simulink model "rlLKAMdl"  (R2019a)
settings: Solver=VariableStepAuto  StartTime=0.0  StopTime=T  RelTol=1e-3
undefined symbols (not defined in the file): Cf, Cr, DiscIntNeverNeededParam, e1_initial, e2_initial, Iz, lf, lr, m, rho, Ts, u_max, u_min, Vx
libraries: rllib x1, simulink x1
settings Model: Creator=The MathWorks, Inc.  LastModifiedBy=The MathWorks, Inc.
settings DataIOCC: ReturnWorkspaceOutputs=off
settings DebuggingCC: ArithmeticOperatorsInVariantConditions=warning
settings SFSimCC: SimUseLocalCustomCode=off
settings RTWCC: RTWUseLocalCustomCode=off
settings CodeAppCC: StateflowObjectComments=on
settings SimscapeCC: SimscapeNormalizeSystem=off

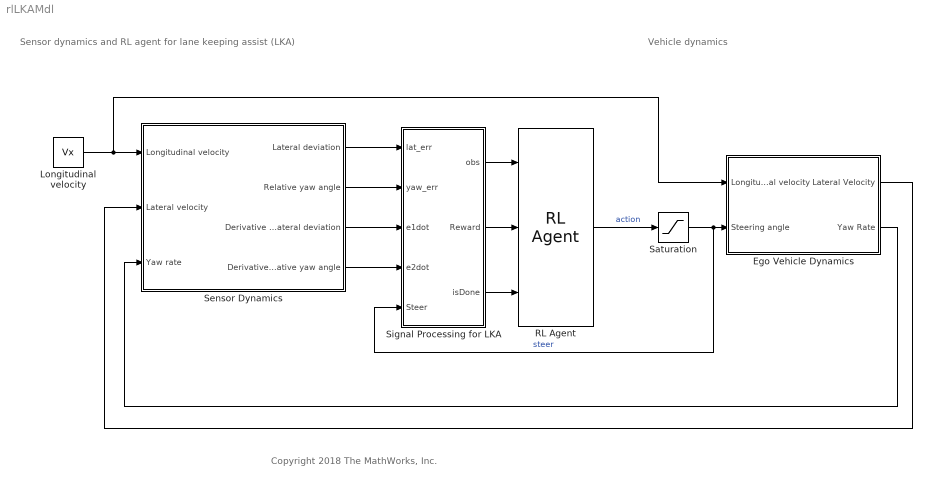
== system rlLKAMdl ==
  note: Vehicle dynamics
  note: Sensor dynamics and RL agent for lane keeping assist (LKA)
  note: Copyright 2018 The MathWorks, Inc.
  Ego Vehicle Dynamics : Subsystem
  Longitudinal velocity : Constant  Value=Vx  SampleTime=Ts
  RL Agent : rllib/RL Agent  Agent=agent  ProvideReward=on  ProvideIsDone=on  ProvideCumRwd=off  TreatAsDirectFeedthrough=on  CollectLoggedSignals=on  CollectModelStates=on
      settings: SourceProductName=Reinforcement Learning Toolbox
  Saturation : Saturate  UpperLimit=u_max  LowerLimit=u_min
  Sensor Dynamics : Subsystem
  "Signal Processing for LKA " : Subsystem
  wires:
  Ego Vehicle Dynamics/2(Yaw Rate) -> Sensor Dynamics/3(Yaw rate)
  Ego Vehicle Dynamics/1(Lateral Velocity) -> Sensor Dynamics/2(Lateral velocity)
  Longitudinal velocity/1 -> Sensor Dynamics/1(Longitudinal velocity), Ego Vehicle Dynamics/1(Longitudinal velocity)
  RL Agent/1 -> Saturation/1  "action"
  Saturation/1 -> "Signal Processing for LKA "/5(Steer), Ego Vehicle Dynamics/2(Steering angle)  "steer"
  Sensor Dynamics/1(Lateral deviation) -> "Signal Processing for LKA "/1(lat_err)
  Sensor Dynamics/2(Relative yaw angle) -> "Signal Processing for LKA "/2(yaw_err)
  "Signal Processing for LKA "/1(obs) -> RL Agent/1
  "Signal Processing for LKA "/2(Reward) -> RL Agent/2
  "Signal Processing for LKA "/3(isDone) -> RL Agent/3
  Sensor Dynamics/3(Derivative of lateral deviation) -> "Signal Processing for LKA "/3("e1dot ")
  Sensor Dynamics/4(Derivative of relative yaw angle) -> "Signal Processing for LKA "/4(e2dot)

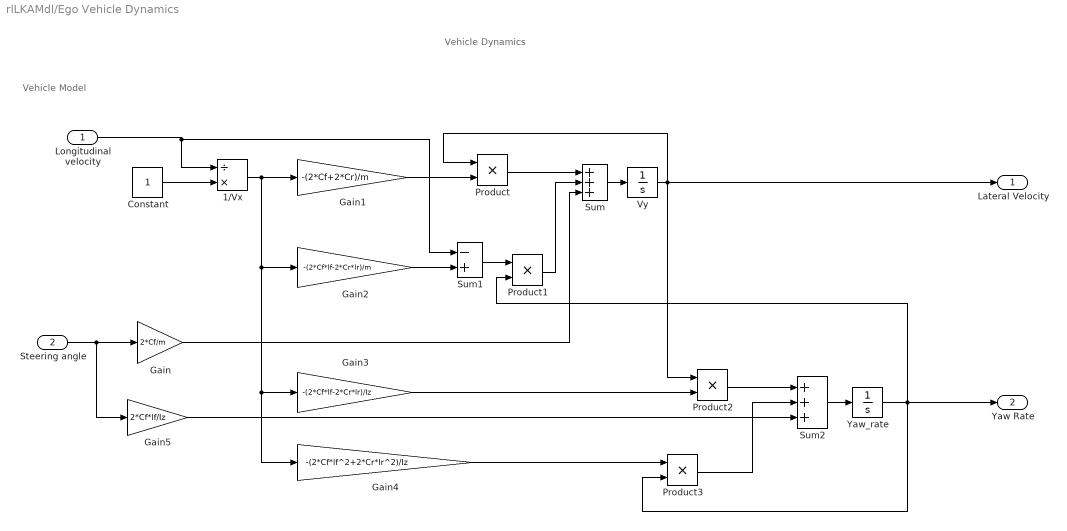
== system rlLKAMdl/Ego Vehicle Dynamics ==
  note: Vehicle Model
  note: Vehicle Dynamics
  Longitudinal velocity : Inport
  Steering angle : Inport  Port=2
  1/Vx : Product  Inputs=/*
  Constant : Constant
  Gain : Gain  Gain=2*Cf/m
  Gain1 : Gain  Gain=-(2*Cf+2*Cr)/m
  Gain2 : Gain  Gain=-(2*Cf*lf-2*Cr*lr)/m
  Gain3 : Gain  Gain=-(2*Cf*lf-2*Cr*lr)/Iz
  Gain4 : Gain  Gain=-(2*Cf*lf^2+2*Cr*lr^2)/Iz
  Gain5 : Gain  Gain=2*Cf*lf/Iz
  Product{,1..3} (4 alike) : Product
  Sum : Sum  Inputs=+++
  Sum1 : Sum  Inputs=-+
  Sum2 : Sum  Inputs=+++
  Vy : Integrator
  "Yaw_rate " : Integrator
  Lateral Velocity : Outport
  Yaw Rate : Outport  Port=2
  wires:
  Sum2/1 -> "Yaw_rate "/1
  Gain2/1 -> Sum1/2
  Gain4/1 -> Product3/1
  Constant/1 -> 1/Vx/2
  Gain3/1 -> Product2/2
  1/Vx/1 -> Gain4/1, Gain3/1, Gain2/1, Gain1/1
  Product2/1 -> Sum2/1
  Product3/1 -> Sum2/2
  Gain5/1 -> Sum2/3
  Sum1/1 -> Product1/1
  "Yaw_rate "/1 -> Product3/2, Yaw Rate/1, Product1/2
  Gain/1 -> Sum/3
  Steering angle/1 -> Gain/1, Gain5/1
  Gain1/1 -> Product/2
  Product/1 -> Sum/1
  Vy/1 -> Product/1, Lateral Velocity/1, Product2/1
  Sum/1 -> Vy/1
  Longitudinal velocity/1 -> Sum1/1, 1/Vx/1
  Product1/1 -> Sum/2

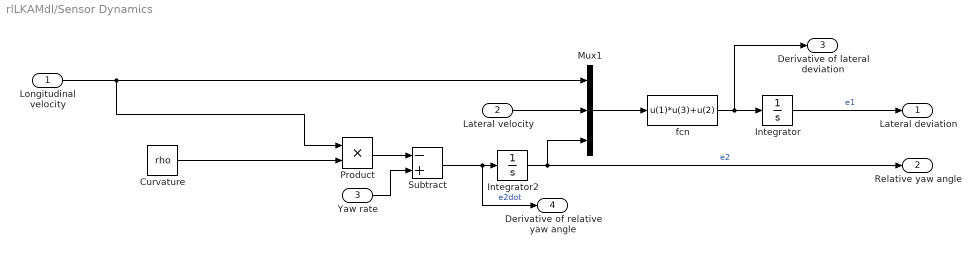
== system rlLKAMdl/Sensor Dynamics ==
  Longitudinal velocity : Inport
  Lateral velocity : Inport  Port=2
  Yaw rate : Inport  Port=3
  Curvature : Constant  Value=rho
  Integrator : Integrator  InitialCondition=e1_initial
  Integrator2 : Integrator  InitialCondition=e2_initial
  Mux1 : Mux  Inputs=[1 1 1]
  Product : Product
  Subtract : Sum  Inputs=-+
  fcn : Fcn  Expr=u(1)*u(3)+u(2)
  Lateral deviation : Outport
  Relative yaw angle : Outport  Port=2
  Derivative of lateral deviation : Outport  Port=3
  Derivative of relative yaw angle : Outport  Port=4
  wires:
  Integrator2/1 -> Relative yaw angle/1, Mux1/3  "e2"
  Mux1/1 -> fcn/1
  fcn/1 -> Derivative of lateral deviation/1, Integrator/1
  Lateral velocity/1 -> Mux1/2
  Integrator/1 -> Lateral deviation/1  "e1"
  Product/1 -> Subtract/1
  Yaw rate/1 -> Subtract/2
  Subtract/1 -> Derivative of relative yaw angle/1, Integrator2/1  "e2dot"
  Longitudinal velocity/1 -> Mux1/1, Product/1
  Curvature/1 -> Product/2

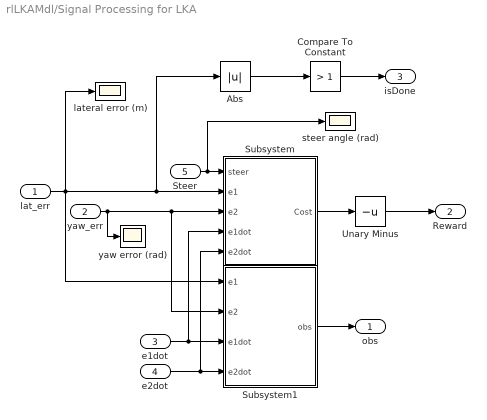
== system rlLKAMdl/Signal Processing for LKA  ==
  lat_err : Inport
  yaw_err : Inport  Port=2
  "e1dot " : Inport  Port=3
  e2dot : Inport  Port=4
  Steer : Inport  Port=5
  Abs : Abs
  Compare To Constant : simulink/Logic and Bit Operations/Compare To Constant  relop=>  const=1  OutDataTypeStr=boolean
  Subsystem : Subsystem
  Subsystem1 : Subsystem
  Unary Minus : UnaryMinus
  lateral error (m) : Scope
  "steer angle (rad) " : Scope
  yaw error (rad) : Scope
  obs : Outport
  Reward : Outport  Port=2
  isDone : Outport  Port=3
  wires:
  Subsystem/1(Cost) -> Unary Minus/1
  Unary Minus/1 -> Reward/1
  lat_err/1 -> Subsystem1/1(e1), Subsystem/2(e1), Abs/1, lateral error (m)/1
  yaw_err/1 -> yaw error (rad)/1, Subsystem1/2(e2), Subsystem/3(e2)
  Abs/1 -> Compare To Constant/1
  Compare To Constant/1 -> isDone/1
  Subsystem1/1(obs) -> obs/1
  "e1dot "/1 -> Subsystem/4(e1dot), Subsystem1/3(e1dot)
  e2dot/1 -> Subsystem/5(e2dot), Subsystem1/4(e2dot)
  Steer/1 -> Subsystem/1(steer), "steer angle (rad) "/1

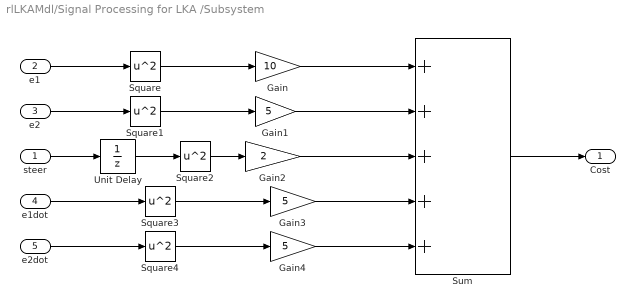
== system rlLKAMdl/Signal Processing for LKA /Subsystem ==
  steer : Inport
  e1 : Inport  Port=2
  e2 : Inport  Port=3
  e1dot : Inport  Port=4
  e2dot : Inport  Port=5
  Gain : Gain  Gain=10
  Gain1 : Gain  Gain=5
  Gain2 : Gain  Gain=2
  Gain3 : Gain  Gain=5
  Gain4 : Gain  Gain=5
  Square{,1..4} (5 alike) : Math  Operator=square  SaturateOnIntegerOverflow=on
  Sum : Sum  Inputs=+++++
  Unit Delay : UnitDelay  SampleTime=-1  HasFrameUpgradeWarning=on
  Cost : Outport
  wires:
  Gain1/1 -> Sum/2
  e1/1 -> Square/1
  e2/1 -> Square1/1
  Sum/1 -> Cost/1
  Gain/1 -> Sum/1
  Square/1 -> Gain/1
  Square1/1 -> Gain1/1
  steer/1 -> Unit Delay/1
  Square2/1 -> Gain2/1
  Gain2/1 -> Sum/3
  Unit Delay/1 -> Square2/1
  Square3/1 -> Gain3/1
  Gain3/1 -> Sum/4
  e1dot/1 -> Square3/1
  e2dot/1 -> Square4/1
  Square4/1 -> Gain4/1
  Gain4/1 -> Sum/5

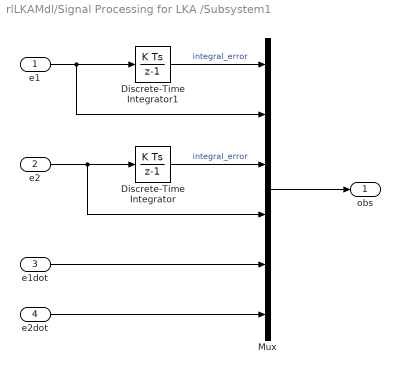
== system rlLKAMdl/Signal Processing for LKA /Subsystem1 ==
  e1 : Inport
  e2 : Inport  Port=2
  e1dot : Inport  Port=3
  e2dot : Inport  Port=4
  Discrete-Time Integrator : DiscreteIntegrator  SampleTime=-1  ICPrevOutput=DiscIntNeverNeededParam  ICPrevScaledInput=DiscIntNeverNeededParam
  Discrete-Time Integrator1 : DiscreteIntegrator  SampleTime=-1  ICPrevOutput=DiscIntNeverNeededParam  ICPrevScaledInput=DiscIntNeverNeededParam
  Mux : Mux  Inputs=6
  obs : Outport
  wires:
  e1/1 -> Mux/2, Discrete-Time Integrator1/1
  Mux/1 -> obs/1
  Discrete-Time Integrator1/1 -> Mux/1  "integral_error"
  e2/1 -> Mux/4, Discrete-Time Integrator/1
  Discrete-Time Integrator/1 -> Mux/3  "integral_error"
  e1dot/1 -> Mux/5
  e2dot/1 -> Mux/6
